simulink library "DoorHndDriver"  (R2022a)
settings: Solver=VariableStepAuto  StartTime=0.0  StopTime=10.0  RelTol=1e-3
settings Model: Creator=DELL  LastModifiedBy=liyun

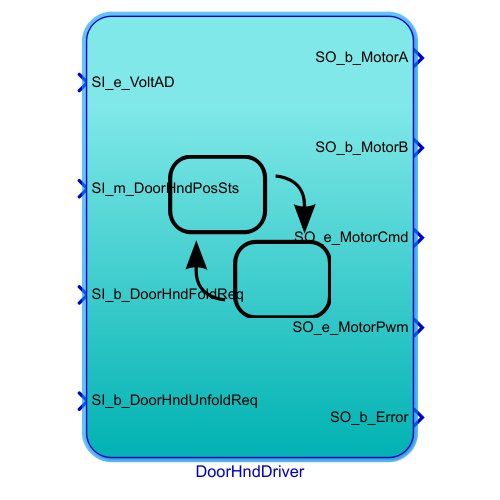
[thumbnail: Simulink's stored preview of the top-level diagram]
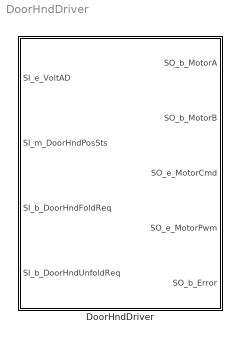
== system DoorHndDriver ==
  DoorHndDriver : Stateflow chart  TreatAsAtomicUnit=on

== stateflow chart DoorHndDriver/DoorHndDriver ==
  note: SO_e_MotorCmd
      | 0: Stop A:0 B:0
      | 1: Unfold A:1 B:0
      | 2: Fold A:0 B:1
  state Drive
    state Idle
      en:
      SO_e_MotorCmd = 0;
      SO_b_MotorA = 0;
      SO_b_MotorB = 0;
      SO_e_MotorPwm = 0;
    state Unfold
      state SoftStartStop
        state Step2
          en:
          /* 保持驱动至门把手展开 */
        state Step1
          /* 软启(线性升压) */
          en:
          SO_e_MotorCmd = 1;
          SO_b_MotorA = 1;
          SO_b_MotorB = 0;
          SO_e_MotorPwm = GetPwm(77); /* 初始电压为7V(AD:77) */
          on every(LinPwmStepTime(30), tick):
          LinPwmUp(SO_e_MotorPwm, GetPwm(139));
          ex:
          SO_e_MotorPwm = GetPwm(139);
        state y = GetPwm(x) [function]
          (default) -> (junction 277) : {y =  (x * 100 / SI_e_VoltAD);}
              | /* 扩大100倍，浮点转整型 */
          (junction 277) -> (junction 285) [order 2]
          (junction 277) -> (junction 283) [order 1] : [y > 100]
              | {y = 100;}
          (junction 285) -> (junction 287)
          (junction 287) -> (junction 283)
          (junction 283) -> (junction 290)
        state Step3
          en:
          /* 检测到门把手展开后进行过驱 */
        state y = LinPwmStepTime(t) [function]
          (default) -> (junction 329) : {y =  t * 10 / (GetPwm(139) - GetPwm(77));}
              | /*  */
          (junction 329) -> (junction 298) : {y = (y + 5) / 10;}
          (junction 298) -> (junction 301) [order 2]
          (junction 298) -> (junction 297) [order 1] : [y == 0]
              | {y = 1;}
          (junction 301) -> (junction 303)
          (junction 303) -> (junction 297)
          (junction 297) -> (junction 306)
        state Step4
          /* 软停(线性降压) */
          en:
          SO_e_MotorPwm = GetPwm(139); /* 初始电压为12V(AD:139) */
          on every(LinPwmStepTime(35), tick):
          LinPwmDown(SO_e_MotorPwm, GetPwm(77));
          ex:
          SO_e_MotorPwm = GetPwm(77);
        state LinPwmUp(x, y) [function]
          (default) -> (junction 334) : [x < y]
              | {x++;}
        state LinPwmDown(x, y) [function]
          (default) -> (junction 340) : [x > y]
              | {x--;}
        (default) -> Drive.Unfold.SoftStartStop.Step1
        Drive.Unfold.SoftStartStop.Step1 -> Drive.Unfold.SoftStartStop.Step2 : after(30, tick)
        Drive.Unfold.SoftStartStop.Step2 -> Drive.Unfold.SoftStartStop.Step3 [order 2] : [SI_m_DoorHndPosSts == Hnd_Unfold] /* 检测门把手是否展开 */
        Drive.Unfold.SoftStartStop.Step3 -> Drive.Unfold.SoftStartStop.Step4 : after(25, tick)
      state Icebreak
        en:
        SL_e_CycleCount = 0;
        state IceBrkWait
          /* 破冰延时 */
          en:
          SO_e_MotorCmd = 0;
          SO_b_MotorA = 0;
          SO_b_MotorB = 0;
          SO_e_MotorPwm = 0;
        state IceBrk
          en:
          SO_e_MotorCmd = 1;
          SO_b_MotorA = 1;
          SO_b_MotorB = 0;
          SO_e_MotorPwm = 100;
        state Check
          en:
          SO_e_MotorCmd = 0;
          SO_b_MotorA = 0;
          SO_b_MotorB = 0;
          SO_e_MotorPwm = 0;
          SL_e_CycleCount++;
        (default) -> IceBrkWait
        IceBrk -> Check [order 2] : after(200, tick)
        IceBrkWait -> IceBrk : after(100, tick)
        Check -> IceBrk [order 2] : [after(100, tick) && ...
            | SL_e_CycleCount < 3]
      state Stop
        en:
        SO_e_MotorCmd = 0;
        SO_b_MotorA = 0;
        SO_b_MotorB = 0;
        SO_e_MotorPwm = 0;
        SO_b_Error = 0;
      (default) -> Drive.Unfold.SoftStartStop
      IceBrk -> Drive.Unfold.Stop [order 1] : [SI_m_DoorHndPosSts == Hnd_Unfold]
          | /* 破冰完成 */
      Drive.Unfold.SoftStartStop.Step4 -> Drive.Unfold.Stop : after(35, tick)
          | /* 正常驱动完成 */
      Drive.Unfold.SoftStartStop.Step2 -> Icebreak [order 1] : after(250, tick) /* 超时进入破冰 */
    state Interrupt1
      /* 折叠打断展开 */
      en:
      SO_e_MotorCmd = 0;
      SO_b_MotorA = 0;
      SO_b_MotorB = 0;
      SO_e_MotorPwm = 0;
    state Interrupt2
      /* 展开打断折叠 */
      en:
      SO_e_MotorCmd = 0;
      SO_b_MotorA = 0;
      SO_b_MotorB = 0;
      SO_e_MotorPwm = 0;
    state Fold
      en:
      state SoftStartStop
        state Step2
          en:
          /* 保持驱动至门把手折叠 */
        state Step1
          en:
          SO_e_MotorCmd = 2;
          SO_b_MotorA = 0;
          SO_b_MotorB = 1;
          SO_e_MotorPwm = GetPwm(77); /* 初始电压为7V(AD:77) */
          on every(LinPwmStepTime(30), tick):
          LinPwmUp(SO_e_MotorPwm, GetPwm(139));
          ex:
          SO_e_MotorPwm = GetPwm(139);
        state y = GetPwm(x) [function]
          (default) -> (junction 393) : {y =  (x * 100 / SI_e_VoltAD);}
          (junction 393) -> (junction 394) [order 2]
          (junction 393) -> (junction 395) [order 1] : [y > 100]
              | {y = 100;}
          (junction 394) -> (junction 396)
          (junction 396) -> (junction 395)
          (junction 395) -> (junction 397)
        state Step3
          en:
          /* 检测到门把手展开后进行过驱 */
        state y = LinPwmStepTime(t) [function]
          (default) -> (junction 408) : {y =  t * 10 / (GetPwm(139) - GetPwm(77));}
          (junction 408) -> (junction 409) : {y = (y + 5) / 10;}
          (junction 409) -> (junction 410) [order 2]
          (junction 409) -> (junction 411) [order 1] : [y == 0]
              | {y = t;}
          (junction 410) -> (junction 412)
          (junction 412) -> (junction 411)
          (junction 411) -> (junction 413)
        state Step4
          en:
          SO_e_MotorPwm = GetPwm(139); /* 初始电压为12V(AD:139) */
          on every(LinPwmStepTime(35), tick):
          LinPwmDown(SO_e_MotorPwm, GetPwm(77));
          ex:
          SO_e_MotorPwm = GetPwm(77);
        state LinPwmUp(x, y) [function]
          (default) -> (junction 425) : [x < y]
              | {x++;}
        state LinPwmDown(x, y) [function]
          (default) -> (junction 430) : [x > y]
              | {x--;}
        (default) -> Drive.Fold.SoftStartStop.Step1
        Drive.Fold.SoftStartStop.Step1 -> Drive.Fold.SoftStartStop.Step2 : after(30, tick)
        Drive.Fold.SoftStartStop.Step2 -> Drive.Fold.SoftStartStop.Step3 [order 2] : [SI_m_DoorHndPosSts == Hnd_Fold]
        Drive.Fold.SoftStartStop.Step3 -> Drive.Fold.SoftStartStop.Step4
      state Stop
        en:
        SO_e_MotorCmd = 0;
        SO_b_MotorA = 0;
        SO_b_MotorB = 0;
        SO_e_MotorPwm = 0;
        SO_b_Error = 0;
      (default) -> Drive.Fold.SoftStartStop
      Drive.Fold.SoftStartStop.Step4 -> Drive.Fold.Stop : after(35, tick)
    (default) -> Idle
    Idle -> Unfold [order 2] : [hasChangedTo(SI_b_DoorHndUnfoldReq, 1)]
    Drive.Unfold.Stop -> Idle
    Unfold -> Interrupt1 : [hasChangedTo(SI_b_DoorHndFoldReq, 1)]
    Interrupt2 -> Unfold : after(10, tick)
    Interrupt1 -> Fold : after(10, tick)
    Fold -> Interrupt2 : [hasChangedTo(SI_b_DoorHndUnfoldReq, 1)]
    Idle -> Fold [order 1] : [hasChangedTo(SI_b_DoorHndFoldReq, 1)]
    Drive.Fold.Stop -> Idle
    Check -> Idle [order 1] : [SL_e_CycleCount >= 3]
        | {SO_b_Error = 1;}
        | /* 破冰达到指定次数，报错 */
    Drive.Fold.SoftStartStop.Step2 -> Idle [order 1] : [after(250, tick)]
        | {SO_b_Error = 1;}
        | /* 超时报错 */
  data: y function_output double; x function_input double; t function_input double; y function_output double; x function_input double; y function_input double; x function_input double; y function_input double; y function_output double; x function_input double; t function_input double; y function_output double; x function_input double; y function_input double; x function_input double; y function_input double; SO_b_MotorA output boolean; SO_b_MotorB output boolean; SO_e_MotorCmd output uint8; SL_e_CycleCount local uint8; SO_e_MotorPwm output uint8; SO_b_Error output boolean; SI_e_VoltAD input uint8; SI_m_DoorHndPosSts input Enum: HndPos_Sts_E; SI_b_DoorHndFoldReq input boolean; SI_b_DoorHndUnfoldReq input boolean
